simulink model "asbCubeSatACS"  (R2019a)
settings: Solver=FixedStepDiscrete  StartTime=0.0  StopTime=10.0  FixedStep=CubeSatTimeStep  RelTol=1e-3  EnableMultiTasking=on
undefined symbols (not defined in the file): gains
libraries: aerolibutil x4, sharedtransform x3, sharedutil x2, asbCubeSatBlockLib x1, simulink x1
settings Model: ExtModeAutoUpdateStatusClock=off  OrderedModelArguments=off  Creator=The MathWorks, Inc.  LastModifiedBy=The MathWorks, Inc.
settings DataIOCC: LimitDataPoints=on  SaveFormat=Array  SaveOutput=off  SignalLogging=off  DSMLogging=off  SaveTime=off  ReturnWorkspaceOutputs=off
settings OptimizationCC: DefaultParameterBehavior=Inlined  OptimizeBlockIOStorage=off  BufferReuse=off  GlobalBufferReuse=off  ExpressionFolding=off  ExpressionDepthLimit=2147483647  LocalBlockOutputs=off  InitFltsAndDblsToZero=on  LifeSpan=inf  OptimizeDataStoreBuffers=off  BusAssignmentInplaceUpdate=off
settings DebuggingCC: ArtificialAlgebraicLoopMsg=none  SolverPrmCheckMsg=warning  FcnCallInpInsideContextMsg=warning  StateNameClashWarn=warning  PregeneratedLibrarySubsystemCodeDiagnostic=none  SFUnexpectedBacktrackingDiag=warning  SFNoUnconditionalDefaultTransitionDiag=warning  SFExecutionAtInitializationDiag=none  ArithmeticOperatorsInVariantConditions=warning
settings HardwareCC: ProdBitPerPointer=32  ProdBitPerSizeT=32  ProdBitPerPtrDiffT=32  ProdLargestAtomicFloat=None  ProdIntDivRoundTo=Undefined  ProdEndianess=Unspecified  ProdWordSize=32  ProdHWDeviceType=32-bit Generic
settings ModelReferenceCC: PropagateSignalLabelsOutOfModel=off
settings SFSimCC: SimUseLocalCustomCode=off
settings RTWCC: RTWUseLocalCustomCode=off
settings CodeAppCC: StateflowObjectComments=on
settings GRTTargetCC: TargetFcnLib=ansi_tfl_tmw.mat  TargetLangStandard=C89/C90 (ANSI)  CombineOutputUpdateFcns=off  GRTInterface=on
settings ConfigComp: CovMetricSettings=dw  CovHtmlReporting=on  CovSaveCumulativeToWorkspaceVar=on  CovSaveSingleToWorkspaceVar=on  CovExternalEMLEnable=off

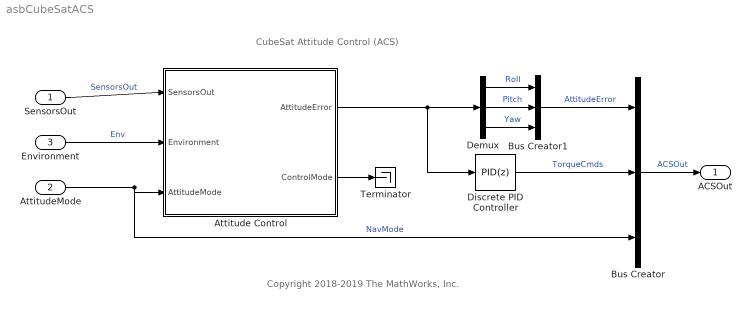
== system asbCubeSatACS ==
  note: Copyright 2018-2019 The MathWorks, Inc.
  note: CubeSat Attitude Control (ACS)
  SensorsOut : Inport  OutDataTypeStr=Bus: StatesOutBus
  AttitudeMode : Inport  Port=2  OutDataTypeStr=double  PortDimensions=1
  Environment : Inport  Port=3  OutDataTypeStr=Bus: EnvBus  PortDimensions=1
  Attitude Control : Subsystem
  Bus Creator : BusCreator  Inputs=3  OutDataTypeStr=Bus: ACSOutBus  NonVirtualBus=on
  Bus Creator1 : BusCreator  Inputs=3  OutDataTypeStr=Bus: AttitudeErrorBus
  Demux : Demux  Outputs=3
  Discrete PID Controller : simulink/Continuous/PID Controller  Controller=PID  Form=Parallel  TimeDomain=Discrete-time  SampleTime=-1  IntegratorMethod=Forward Euler  FilterMethod=Forward Euler  ControllerParametersSource=internal  P=gains.Kp  I=gains.Ki  D=gains.Kd  UseFilter=off  N=1000  TunerSelectOption=Transfer Function Based (PID Tuner App)  InitialConditionSource=internal  InitialConditionForIntegrator=0  InitialConditionForFilter=0  DifferentiatorICPrevScaledInput=0  ExternalReset=none  TrackingMode=off  Kt=1  LimitOutput=off  UpperSaturationLimit=inf  LowerSaturationLimit=-inf  LinearizeAsGain=off  AntiWindupMode=none  Kb=1  POutMin=[]  POutMax=[]  IOutMin=[]  IOutMax=[]  DOutMin=[]  DOutMax=[]  NOutMin=[]  NOutMax=[]  SumOutMin=[]  SumOutMax=[]  SaturationOutMin=[]  SaturationOutMax=[]  PParamMin=[]  PParamMax=[]  IParamMin=[]  IParamMax=[]  DParamMin=[]  DParamMax=[]  NParamMin=[]  NParamMax=[]  KbParamMin=[]  KbParamMax=[]  KtParamMin=[]  KtParamMax=[]  KbOutMin=[]  KbOutMax=[]  KtOutMin=[]  KtOutMax=[]  IntegratorOutMin=[]  IntegratorOutMax=[]  FilterOutMin=[]  FilterOutMax=[]  SumI1OutMin=[]  SumI1OutMax=[]  SumI2OutMin=[]  SumI2OutMax=[]  SumI3OutMin=[]  SumI3OutMax=[]  SumI4OutMin=[]  SumI4OutMax=[]  SumDOutMin=[]  SumDOutMax=[]  DifferentiatorOutMin=[]  DifferentiatorOutMax=[]  FilterDiffOutCoefMin=[]  FilterDiffOutCoefMax=[]  ReciprocalOutMin=[]  ReciprocalOutMax=[]  SumDenOutMin=[]  SumDenOutMax=[]  SumNumOutMin=[]  SumNumOutMax=[]  DivideOutMin=[]  DivideOutMax=[]  IntegratorContinuousStateAttributes=''  IntegratorStateMustResolveToSignalObject=off  IntegratorRTWStateStorageClass=Auto  FilterContinuousStateAttributes=''  FilterStateMustResolveToSignalObject=off  FilterRTWStateStorageClass=Auto  ParallelPVariant=InternalParameters  IdealPVariant=Disabled  IVariant=InternalParameters  DVariant=InternalParameters  IntegratorVariant=Discrete  SatVariant=Disabled  AWVariant=Passthrough  PCopyVariant=Disabled  TRVariant=Disabled  FdbkBlocksVariant=Forward  IdealPFdbkVariant=Disabled  SatFdbkVariant=Disabled  DerivativeFilterVariant=Differentiator  NVariant=Passthrough  NCopyVariant=Disabled_SignalSpec  FilterICVariant=InternalICsDifferentiator  IntegratorICVariant=InternalICs  ExternalResetVariant=Disabled  TRSumVariant=Passthrough  SumFdbkVariant=Disabled  SumVariant=Sum_PID
  Terminator : Terminator
  ACSOut : Outport  OutDataTypeStr=Bus: ACSOutBus  PortDimensions=1  BusOutputAsStruct=on
  wires:
  Demux/1 -> Bus Creator1/1  "Roll"
  AttitudeMode/1 -> Attitude Control/3("AttitudeMode "), Bus Creator/3  "NavMode"
  Demux/2 -> Bus Creator1/2  "Pitch"
  SensorsOut/1 -> Attitude Control/1("SensorsOut ")  "SensorsOut"
  Bus Creator1/1 -> Bus Creator/1  "AttitudeError"
  Demux/3 -> Bus Creator1/3  "Yaw"
  Discrete PID Controller/1 -> Bus Creator/2  "TorqueCmds"
  Bus Creator/1 -> ACSOut/1  "ACSOut"
  Attitude Control/1(AttitudeError) -> Discrete PID Controller/1, Demux/1
  Attitude Control/2(" ControlMode") -> Terminator/1
  Environment/1 -> Attitude Control/2(Environment)  "Env"

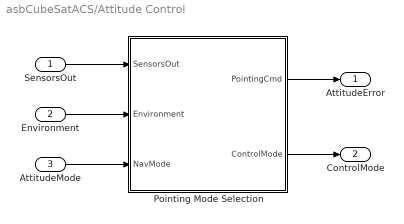
== system asbCubeSatACS/Attitude Control ==
  "SensorsOut " : Inport  OutDataTypeStr=Bus: StatesOutBus
  Environment : Inport  Port=2
  "AttitudeMode " : Inport  Port=3
  Pointing Mode Selection : Stateflow chart  TreatAsAtomicUnit=on
  AttitudeError : Outport
  " ControlMode" : Outport  Port=2
  wires:
  "SensorsOut "/1 -> Pointing Mode Selection/1(SensorsOut)
  Pointing Mode Selection/2(ControlMode) -> " ControlMode"/1
  "AttitudeMode "/1 -> Pointing Mode Selection/3(NavMode)
  Environment/1 -> Pointing Mode Selection/2(Environment)
  Pointing Mode Selection/1(PointingCmd) -> AttitudeError/1

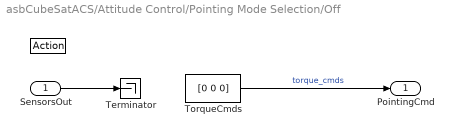
== system asbCubeSatACS/Attitude Control/Pointing Mode Selection/Off ==
  SensorsOut : Inport  OutDataTypeStr=Bus: StatesOutBus
  " " : ActionPort
      settings: CopyFcn=Stateflow.SLINSF.SimulinkMan.removeBlockPreDeleteFcn  PreDeleteFcn=Stateflow.SLINSF.SimulinkMan.unsafePredeleteFcn
  Terminator : Terminator
  TorqueCmds : Constant  Value=[0 0 0]
  PointingCmd : Outport
  wires:
  SensorsOut/1 -> Terminator/1
  TorqueCmds/1 -> PointingCmd/1  "torque_cmds"

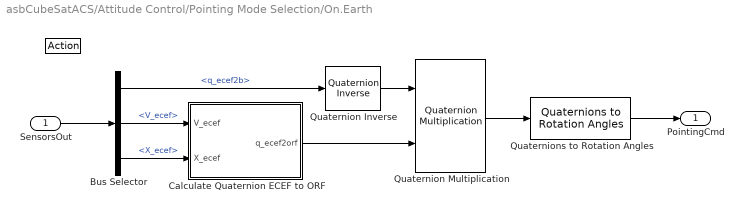
== system asbCubeSatACS/Attitude Control/Pointing Mode Selection/On.Earth ==
  SensorsOut : Inport  OutDataTypeStr=Bus: StatesOutBus
  " " : ActionPort
      settings: CopyFcn=Stateflow.SLINSF.SimulinkMan.removeBlockPreDeleteFcn  PreDeleteFcn=Stateflow.SLINSF.SimulinkMan.unsafePredeleteFcn
  Bus Selector : BusSelector  OutputSignals=q_ecef2b,V_ecef,X_ecef
  Calculate Quaternion ECEF to ORF : Subsystem
  Quaternion Inverse : aerolibutil/Quaternion Inverse
      settings: SourceProductName=Aerospace Blockset
  Quaternion Multiplication : aerolibutil/Quaternion Multiplication
  Quaternions to Rotation Angles : sharedtransform/Quaternions to Rotation Angles  rotationOrder=XYZ  aMode=aMode
      settings: SourceProductBaseCode=AE
  PointingCmd : Outport
  wires:
  Quaternions to Rotation Angles/1 -> PointingCmd/1
  Quaternion Inverse/1 -> Quaternion Multiplication/1
  Quaternion Multiplication/1 -> Quaternions to Rotation Angles/1
  Calculate Quaternion ECEF to ORF/1(q_ecef2orf) -> Quaternion Multiplication/2
  Bus Selector/1 -> Quaternion Inverse/1  "<q_ecef2b>"
  Bus Selector/3 -> Calculate Quaternion ECEF to ORF/2(X_ecef)  "<X_ecef>"
  Bus Selector/2 -> Calculate Quaternion ECEF to ORF/1(V_ecef)  "<V_ecef>"
  SensorsOut/1 -> Bus Selector/1

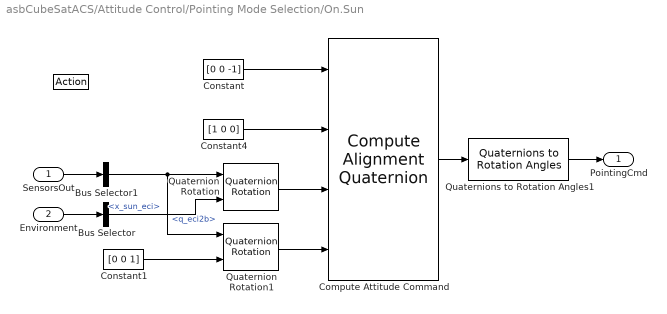
== system asbCubeSatACS/Attitude Control/Pointing Mode Selection/On.Sun ==
  SensorsOut : Inport  OutDataTypeStr=Bus: StatesOutBus
  Environment : Inport  Port=2  OutDataTypeStr=Bus: EnvBus
  " " : ActionPort
      settings: CopyFcn=Stateflow.SLINSF.SimulinkMan.removeBlockPreDeleteFcn  PreDeleteFcn=Stateflow.SLINSF.SimulinkMan.unsafePredeleteFcn
  Bus Selector : BusSelector  OutputSignals=x_sun_eci
  Bus Selector1 : BusSelector  OutputSignals=q_eci2b
  Compute Attitude Command : asbCubeSatBlockLib/Axes Transformations/Attitude Conversion/Compute Alignment Quaternion  SystemSampleTime=-1
  Constant : Constant  Value=[0 0 -1]
  Constant1 : Constant  Value=[0 0 1]
  Constant4 : Constant  Value=[1 0 0]
  Quaternion Rotation : aerolibutil/Quaternion Rotation
  Quaternion Rotation1 : aerolibutil/Quaternion Rotation
  Quaternions to Rotation Angles1 : sharedtransform/Quaternions to Rotation Angles  rotationOrder=XYZ  aMode=aMode
      settings: SourceProductBaseCode=AE
  PointingCmd : Outport
  wires:
  Compute Attitude Command/1 -> Quaternions to Rotation Angles1/1
  Constant1/1 -> Quaternion Rotation1/2
  Bus Selector/1 -> Quaternion Rotation/2  "<x_sun_eci>"
  Bus Selector1/1 -> Quaternion Rotation1/1, Quaternion Rotation/1  "<q_eci2b>"
  Constant4/1 -> Compute Attitude Command/2
  Constant/1 -> Compute Attitude Command/1
  SensorsOut/1 -> Bus Selector1/1
  Environment/1 -> Bus Selector/1
  Quaternion Rotation/1 -> Compute Attitude Command/3
  Quaternion Rotation1/1 -> Compute Attitude Command/4
  Quaternions to Rotation Angles1/1 -> PointingCmd/1

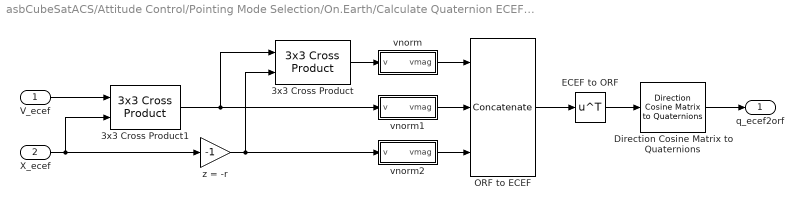
== system asbCubeSatACS/Attitude Control/Pointing Mode Selection/On.Earth/Calculate Quaternion ECEF to ORF ==
  V_ecef : Inport
  X_ecef : Inport  Port=2
  3x3 Cross Product : sharedutil/3x3 Cross Product  aMode=aMode
      settings: SourceProductBaseCode=AE
  3x3 Cross Product1 : sharedutil/3x3 Cross Product  aMode=aMode
      settings: SourceProductBaseCode=AE
  Direction Cosine Matrix to Quaternions : sharedtransform/Direction Cosine Matrix  to Quaternions  aMode=0  action=None  tolerance=eps(2)
      settings: SourceProductName=Aerospace Blockset  SourceProductBaseCode=AE
  ECEF to ORF : Math  Operator=transpose  SaturateOnIntegerOverflow=on
  ORF to ECEF : Concatenate  NumInputs=3  Mode=Multidimensional array  ConcatenateDimension=2
  vnorm : Subsystem
      mask Display: disp('v norm')
  vnorm1 : Subsystem
      mask Display: disp('v norm')
  vnorm2 : Subsystem
      mask Display: disp('v norm')
  z = -r : Gain  Gain=-1
  q_ecef2orf : Outport
  wires:
  Direction Cosine Matrix to Quaternions/1 -> q_ecef2orf/1
  3x3 Cross Product1/1 -> 3x3 Cross Product/1, vnorm1/1(v)
  X_ecef/1 -> 3x3 Cross Product1/2, z = -r/1
  3x3 Cross Product/1 -> vnorm/1(v)
  z = -r/1 -> 3x3 Cross Product/2, vnorm2/1(v)
  V_ecef/1 -> 3x3 Cross Product1/1
  vnorm1/1(vmag) -> ORF to ECEF/2
  vnorm2/1(vmag) -> ORF to ECEF/3
  vnorm/1(vmag) -> ORF to ECEF/1
  ORF to ECEF/1 -> ECEF to ORF/1
  ECEF to ORF/1 -> Direction Cosine Matrix to Quaternions/1

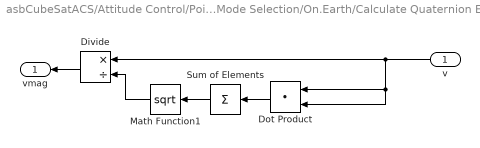
== system asbCubeSatACS/Attitude Control/Pointing Mode Selection/On.Earth/Calculate Quaternion ECEF to ORF/vnorm ==
  v : Inport
  Divide : Product  Inputs=*/
  Dot Product : DotProduct  InputSameDT=on  OutDataTypeStr=Inherit: Inherit via internal rule
  Math Function1 : Math  Operator=sqrt  SaturateOnIntegerOverflow=on
  Sum of Elements : Sum  Inputs=+
  vmag : Outport
  wires:
  Dot Product/1 -> Sum of Elements/1
  Sum of Elements/1 -> Math Function1/1
  Math Function1/1 -> Divide/2
  v/1 -> Divide/1, Dot Product/2, Dot Product/1
  Divide/1 -> vmag/1

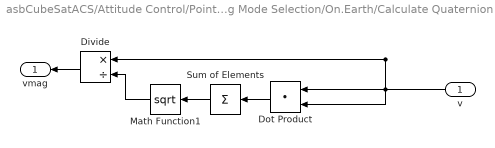
== system asbCubeSatACS/Attitude Control/Pointing Mode Selection/On.Earth/Calculate Quaternion ECEF to ORF/vnorm1 ==
  v : Inport
  Divide : Product  Inputs=*/
  Dot Product : DotProduct  InputSameDT=on  OutDataTypeStr=Inherit: Inherit via internal rule
  Math Function1 : Math  Operator=sqrt  SaturateOnIntegerOverflow=on
  Sum of Elements : Sum  Inputs=+
  vmag : Outport
  wires:
  Divide/1 -> vmag/1
  v/1 -> Dot Product/1, Dot Product/2, Divide/1
  Math Function1/1 -> Divide/2
  Sum of Elements/1 -> Math Function1/1
  Dot Product/1 -> Sum of Elements/1

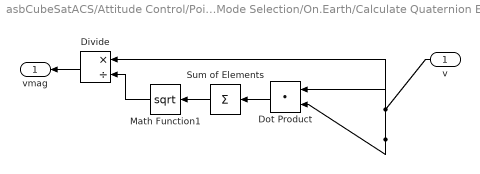
== system asbCubeSatACS/Attitude Control/Pointing Mode Selection/On.Earth/Calculate Quaternion ECEF to ORF/vnorm2 ==
  v : Inport
  Divide : Product  Inputs=*/
  Dot Product : DotProduct  InputSameDT=on  OutDataTypeStr=Inherit: Inherit via internal rule
  Math Function1 : Math  Operator=sqrt  SaturateOnIntegerOverflow=on
  Sum of Elements : Sum  Inputs=+
  vmag : Outport
  wires:
  Dot Product/1 -> Sum of Elements/1
  Sum of Elements/1 -> Math Function1/1
  Math Function1/1 -> Divide/2
  v/1 -> Divide/1, Dot Product/2, Dot Product/1
  Divide/1 -> vmag/1

== stateflow chart asbCubeSatACS/Attitude Control/Pointing Mode Selection ==
  state On
    state Transition
    state Earth
    state Sun
    (default) -> Transition
    Transition -> Sun [order 2] : [NavMode == 2]
        | {ControlMode = 2;}
    Sun -> Transition : [NavMode == 1]
        | {ControlMode = 1;}
    Transition -> Earth [order 1] : [NavMode == 1]
        | {ControlMode = 2;}
    Earth -> Transition : [NavMode == 2]
        | {ControlMode = 1;}
  state Off
  (default) -> Off
  Off -> On : [NavMode ~= 0]
      | {ControlMode = 1;}
  On -> Off : [NavMode == 0]
      | {ControlMode = 0;}
  data: sf_internal_action_state_placeholder_data local double size=1 =0; sf_internal_action_state_placeholder_data local double size=1 =0; sf_internal_action_state_placeholder_data local double size=1 =0; SensorsOut input Bus: StatesOutBus; Environment input; NavMode input; PointingCmd output =[0 0 0]'; ControlMode output
